simulink model "hug3vertical_from_github"  (R2021a)
settings: Solver=ode45  StartTime=0.0  StopTime=100  FixedStep=1  RelTol=1e-3
settings Model: Creator=daoist  LastModifiedBy=daoist

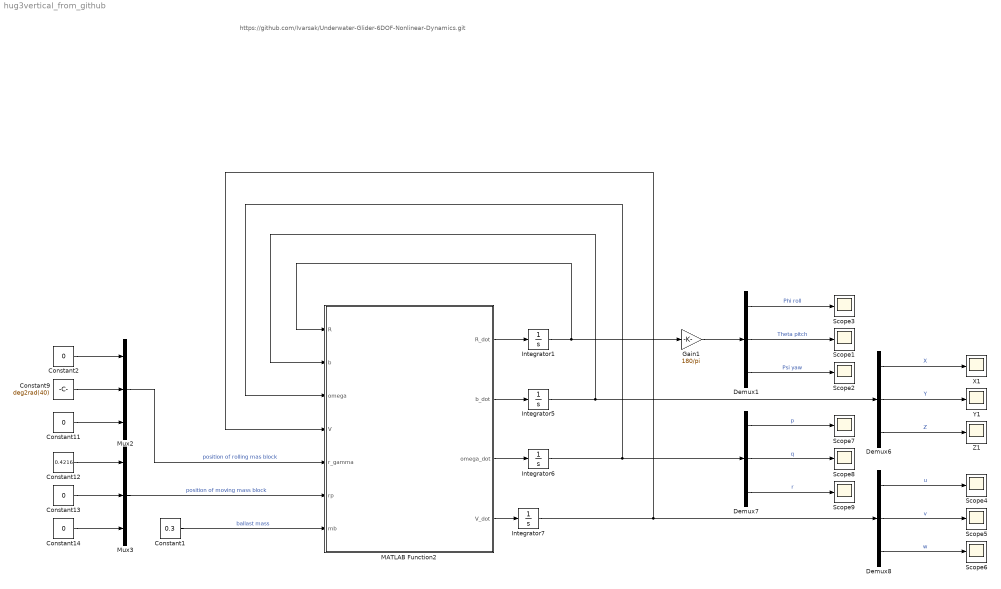
== system hug3vertical_from_github ==
  note: https://github.com/Ivarsak/Underwater-Glider-6DOF-Nonlinear-Dynamics.git
  Constant1 : Constant  Value=0.3
  Constant{2,11,13..14} (4 alike) : Constant  Value=0
  Constant12 : Constant  Value=0.4216
  Constant9 : Constant  Value=deg2rad(40)
  Demux{1,6..8} (4 alike) : Demux  Outputs=3
  Gain1 : Gain  Gain=180/pi
  Integrator1 : Integrator  InitialCondition=[0 0 0]
  Integrator5 : Integrator  InitialCondition=[0 0 0]
  Integrator6 : Integrator  InitialCondition=[0 0 0]
  Integrator7 : Integrator  InitialCondition=[0.01 0 0]
  MATLAB Function2 : MATLAB Function  TreatAsAtomicUnit=on
  Mux2 : Mux  Inputs=3
  Mux3 : Mux  Inputs=3
  Scope{1..9} (9 alike) : Scope
  X1 : Scope
  Y1 : Scope
  Z1 : Scope
  wires:
  Mux3/1 -> MATLAB Function2/6(rp)  "position of moving mass block"
  Mux2/1 -> MATLAB Function2/5(r_gamma)  "position of rolling mas block"
  Constant14/1 -> Mux3/3
  Constant13/1 -> Mux3/2
  Constant9/1 -> Mux2/2
  Constant1/1 -> MATLAB Function2/7(mb)  "ballast mass"
  Constant11/1 -> Mux2/3
  Constant2/1 -> Mux2/1
  Constant12/1 -> Mux3/1
  Gain1/1 -> Demux1/1
  Demux7/3 -> Scope9/1  "r"
  Demux7/1 -> Scope7/1  "p"
  MATLAB Function2/4(V_dot) -> Integrator7/1
  Demux7/2 -> Scope8/1  "q"
  Integrator6/1 -> Demux7/1, MATLAB Function2/3(omega)
  Integrator5/1 -> Demux6/1, MATLAB Function2/2(b)
  Demux6/2 -> Y1/1  "Y"
  Demux6/3 -> Z1/1  "Z"
  Integrator7/1 -> Demux8/1, MATLAB Function2/4(V)
  MATLAB Function2/3(omega_dot) -> Integrator6/1
  Demux6/1 -> X1/1  "X"
  Demux1/1 -> Scope3/1  "Phi roll"
  Demux1/2 -> Scope1/1  "Theta pitch"
  Demux1/3 -> Scope2/1  "Psi yaw"
  MATLAB Function2/2(b_dot) -> Integrator5/1
  MATLAB Function2/1(R_dot) -> Integrator1/1
  Integrator1/1 -> Gain1/1, MATLAB Function2/1(R)
  Demux8/3 -> Scope6/1  "w"
  Demux8/1 -> Scope4/1  "u"
  Demux8/2 -> Scope5/1  "v"

== matlab function hug3vertical_from_github/MATLAB Function2 ==
  data: R input; b input; omega input; V input; r_gamma input; rp input; mb input; R_dot output; b_dot output; omega_dot output; V_dot output
function [ R_dot, b_dot, omega_dot, V_dot] =Glider_function_vectorial(R, b, omega, V, r_gamma, rp, mb )
% Gamma_dot, rp1_dot, mb_dot

function [s] = S(x1,x2,x3)
        s = [0 -x3 x2;
             x3 0 -x1;
             -x2 x1 0];
end
e1 = [1 0 0]';                     %Body frame unit vector along x
e2 = [0 1 0]';                     %Body frame unit vector along y
e3 = [0 0 1]';                     %Body frame unit vector along z

I3 = eye(3);                      %Identity matrix (3x3)

%% Masses

% 静质量
m_s = 54.28;                     %Hull mass [Kg]
% 质心调节质量块
m_p = 11;                        %Longitiudal and lateral moving mass [kg]
% 浮力
m = 65.28;                       %Displacement of fluid mass [Kg]
% 浮力调节质量
m_b = 0.5;                       %Net buoyancy mass [kg]
m_t = m_s + m_p;                 %Total mass
g = 9.81;                        %Gravity accleration

% 航行器对体坐标系的转动惯量 Jx Jy Jz
I_s = diag([0.60 15.27 15.32]);  %Inertia of static block/hull
I_rm = diag([0.02 10.16 0.17]);  %Inertia of movable block mass
Rr = 0.014;                      %Movable mass offset [m]
%% Added mass Matrix M_A

% 附加惯性质量、附加转动惯量
% 在纵向分析时，认为机体是椭球体，有三个对称面，附加静惯性矩=0（刚体平移与转动的耦合项）
% 该项仅与流体动能有关
M_A = [diag([1.48 49.58 10.18]) zeros(3);
       zeros(3) diag([0.53 7.88 10.18]) ];

   
%% Hydrodynamic coefficients for forces and moments
% 水动力与水动力力矩系数
KD0 = 7.19;                     %Coefficient of Drag force [X] 
KD = 386.29;                    %Coefficient of Drag force [X] 
KL0 = -0.36;                    %Coefficient of Lift force [Z] 
K_alpha = 440.99;               %Coefficient of Lift force [Z] ?KL

KMR = -58.27;                   %Coefficient of moment [K]
Kp = -19.83;                    %Coefficient of moment [K]

KM0 = 0.28;                     %Coefficient of moment [M] 
KM = -65.84;                    %Coefficient of moment [M]
Kq = -205.64;                   %Coefficient of moment [M] 

KMY = 34.10;                    %Coefficient of moment [N]
Kr = -389.30;                   %Coefficient of moment [N]
K_beta = -115.65;               %Coefficient of Sideforce  [Y]  总侧滑力矩系数
%% RK ODE solver


%Initalizing ballast mass and mass block positions

Gamma_d = deg2rad(40);              %Servo Angle [Rad]
% Gamma_d = 0; % 质量块偏转角度
rp1_d = 0.4216;                     %Moving mass block position [m]
mb_d = 0.3;                         %Ballast mass [Kg]

%Vectors to store ODE data in

%% 
%R(1) = Phi (roll), R(2) = Theta (pitch), R(3) = Psi (yaw)
%b(1) = x, b(2) = y, b(3) = z
%omega(1) = p, omega(2) = q, omega(3) = r
%V(1) = V1, V(2) = V2, V(3) = V3 in body frame
%r_gamma(1) = 0, r_gamma(2) = Gamma, r_gamma(3) = 0 position of rolling mass block
%rp(1) = rp1, rp(2) = rp2, rp(3) = rp3 position of moving mass block
%mb -> ballast mass
mb = mb_d;
u = V(1);     %Sway velocity 
v = V(2);     %Heave velocity
w = V(3);     %Surge velocity 
p = omega(1); %Angular velocity around roll angle, Phi
q = omega(2); %Angular velocity around pitch angle, Theta
r = omega(3); %Angular velocity around yaw angle, Psi
u_gamma = [0 0 0]';
u_mp    = [0 0 0]';
u_mb    = 0;

tau = [0 0 0 u_gamma(2) u_mp(1) 0]';  %Control inputs

m_t = mb + m_p + m_s;
 
%% Kinematics

% Rotation matrix to map the Euler Angle attitudes
% 体坐标系中角速度向惯性坐标系中角速度转换
n_1 = [1 sin(R(1))*tan(R(2)) cos(R(1))*tan(R(2));
       0    cos(R(1))            -sin(R(1));
       0 sin(R(1))*sec(R(2))    cos(R(1))*sec(R(2))];
   

%Rotation matrix to map the translational velocities in the body frame
% 体坐标系中平直速度向惯性坐标系中平直速度的转换
n_2 = [cos(R(3))*cos(R(2))    (-sin(R(3))*cos(R(1)) + cos(R(3))*sin(R(2))*sin(R(1))) (sin(R(3))*sin(R(1)) + cos(R(3))*cos(R(1))*sin(R(2)));
     sin(R(3))*cos(R(2))    (cos(R(3))*cos(R(1)) + sin(R(1))*sin(R(2))*sin(R(3)))  (-cos(R(3))*sin(R(1)) + sin(R(2))*sin(R(3))*cos(R(1)));
     -sin(R(2))            cos(R(2))*sin(R(1))                                 cos(R(2))*cos(R(1))];


%Inertia matrix for the rolling mass
R_x = [1 0 0;
       0 cos(r_gamma(2)) -sin(r_gamma(2));
       0 sin(r_gamma(2)) cos(r_gamma(2))];
   
%% Computing Hydrodynamic Damping Matrix D(v)
% 速度坐标系中，水动力计算
   v_r = sqrt(u^2 + v^2 + w^2);
   
   Alpha = atan(w/u);                     %Angle of attack
   Beta  = asin(v/v_r);                   %Sideslip angle
   
   X = (KD0 + (KD*(Alpha^2)))*v_r^2;       %Drag force
   Y = (K_beta*Beta)*v_r^2;                %Sideforce
   Z = (KL0 + K_alpha*Alpha)*v_r^2;        %Lift force
   
   K = (KMR*Beta + Kp*p)*v_r^2;            %Roll Moment
   M = (KM0 + KM*Alpha + Kq*q)*v_r^2;      %Pitch Moment
   N = (KMY*Beta + Kr*r)*v_r^2;            %Yaw Moment
   
   F_hy = [X -Y Z]';                        %Total Hydrodynamic force in flow frame
   M_hy = [-K -M -N]';                      %Total hydrodynamic moment in flow frame

   
 %Rotation matrix from the flow frame to body frame
 % 速度坐标系向体坐标系转换，力与力矩
    R_BF = [cos(Alpha)*cos(Beta) -cos(Alpha)*sin(Beta) -sin(Alpha);
            sin(Beta) cos(Beta) 0;
            sin(Alpha)*cos(Beta) -sin(Alpha)*sin(Beta) cos(Alpha)];
     
  % Damping Matrix
   D_v = [R_BF*F_hy; R_BF*M_hy];
   

 %% Computing Restoring Forces
 % 恢复力
F_G = [0 0 m_t*g]';      %Gravitational force in NED {n}
F_B = [0 0 -m*g]';       %Buoyant force in NED {n}

%Computing the CG and CB vectors in body-frame {b}
% 重心 浮心在体坐标系中向量

% 质量块、浮力装置质量、机体质量的坐标（在体坐标系中）
r_mp = rp(1)*e1 + Rr*(cos(r_gamma(2) + pi/2)*e2 + sin(r_gamma(2) + pi/2)*e3); %Position of moving mass/rolling mass block 公式9
% r_mp = rp1_d*e1 ;
r_mb = [0 0 0]';                                                              %Position of internal ballast tank (fixed)
r_s = [-0.0814 0 0.0032]';                                                    %Position of static mass (fixed)

% 由上述质心得到整体的质心、浮心（体坐标系原点在浮心）
r_CB = [0 0 0]';                             %CB vector. Coincides with body-fixed origin O_{b} = [0,0,0]^T
r_CG = (r_mp*m_p + r_mb*m_b + r_s*m_s)/m_t;   %CG vector. Which is offset from CB = [0,0,0] in the body frame {b}

rx_CG = r_CG(1);                             %CG in x-axis
ry_CG = r_CG(2);                             %CG in y-axis
rz_CG = r_CG(3);                             %CG in z-axis

%Computing the restoring terms g(n) in the body-frame {b}
% 计算得到体坐标系中，质量引起的直力与力矩（由公式4 5 反推）
% n_2'由惯性向体坐标系转换
 G_n = -[n_2'*(F_G + F_B);
        cross(r_CG, n_2'*F_G) + cross(r_CB, n_2'*F_B)];
           
%% Computing Rigid-Body Dynamics
 %-------------------------------------------------------------------------------------------------------------------
 %------------------------------------------------------------------------------------------------------------------- 
 %Computing the Total System Inertia Matrix - M
 % 公式15 中的M
 % I_mp : Ir(y); I_rm: Ir(0)
 I_mp = (R_x'*I_rm*R_x);                    %Inertia of the moving/rolling mass block m_p about CB/CO
 I_rb = I_s + I_mp;                         %Total inertia about CB
 
 M_rb = [m_t*I3 -m_t*S(rx_CG,ry_CG,rz_CG);  %Rigid-Body system Inertia Matrix
         m_t*S(rx_CG,ry_CG,rz_CG) I_rb];
     
 M = M_rb + M_A;                            %Total System Inertia Matrix  
 %-------------------------------------------------------------------------------------------------------------------
 %-------------------------------------------------------------------------------------------------------------------
 % Computing the Coriolis and Centripetal Matrix C(v)
 
 IO = I_rb*omega;      
 % 柯氏力与柯氏力矩 矩阵
 C_v = [zeros(3) (-m_t*S(u,v,w) - m_t*S(p,q,r)*S(rx_CG,ry_CG,rz_CG));
        (-m_t*S(u,v,w) + m_t*S(rx_CG,ry_CG,rz_CG)*S(p,q,r)) -S(IO(1), IO(2), IO(3))];
    

%% Computing the Equations of Motion
% 公式16 19
 v_dot = inv(M)*(-D_v - C_v*[u v w p q r]' - G_n + tau); %6DOF dynamics
 
R_dot =     n_1*omega;                         %Kinematic equation  
b_dot =     n_2*V;                             %Kinematic equation 
V_dot =     [v_dot(1) v_dot(2) v_dot(3)]';      %Dynamic equation 
omega_dot = [v_dot(4) v_dot(5) v_dot(6)]';      %Dyamic equation 

%Control inputs

% rp1_dot =   u_mp;         
% Gamma_dot = u_gamma;      
% mb_dot =    u_mb;        
% 
% 
% %Return vector for the ODE45 solver
% T =[R_dot' b_dot' omega_dot' V_dot' Gamma_dot' rp1_dot' mb_dot']'; 

    
end
